simulink model "pure_linearization"  (R2023a)
settings: Solver=VariableStepAuto  StartTime=0.0  StopTime=5  RelTol=1e-3
settings Model: Creator=szymo  LastModifiedBy=szymo

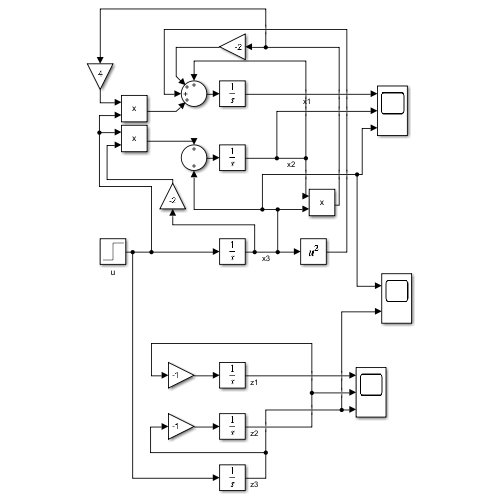
[thumbnail: Simulink's stored preview of the top-level diagram]
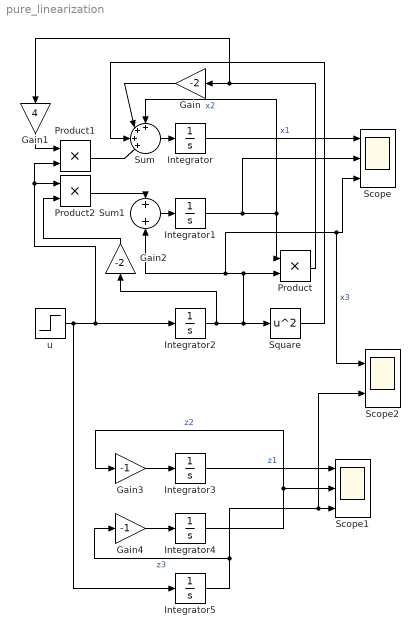
== system pure_linearization ==
  Gain : Gain  Gain=-2
  Gain1 : Gain  Gain=4
  Gain2 : Gain  Gain=-2
  Gain3 : Gain  Gain=-1
  Gain4 : Gain  Gain=-1
  Integrator{,1..5} (6 alike) : Integrator
  Product : Product
  Product1 : Product
  Product2 : Product
  Scope : Scope  NumInputPorts=3
  Scope1 : Scope  NumInputPorts=3
  Scope2 : Scope  NumInputPorts=2
  Square : Math  Operator=square
  Sum : Sum  Inputs=++++|
  Sum1 : Sum
  u : Step  Time=0  SampleTime=0
  wires:
  Sum/1 -> Integrator/1
  Integrator1/1 -> Scope/2, Product/1, Sum/1  "x2"
  Integrator/1 -> Scope/1  "x1"
  Integrator2/1 -> Gain2/1, Scope2/1, Scope/3, Sum1/2, Product/2, Square/1  "x3"
  Product/1 -> Gain1/1, Gain/1
  Gain/1 -> Sum/2
  Square/1 -> Sum/3
  Sum1/1 -> Integrator1/1
  u/1 -> Integrator5/1, Product2/1, Product1/2, Integrator2/1
  Product1/1 -> Sum/4
  Gain1/1 -> Product1/1
  Gain2/1 -> Product2/2
  Product2/1 -> Sum1/1
  Integrator3/1 -> Scope1/1  "z1"
  Integrator4/1 -> Scope1/2, Gain3/1  "z2"
  Integrator5/1 -> Scope2/2, Scope1/3, Gain4/1  "z3"
  Gain4/1 -> Integrator4/1
  Gain3/1 -> Integrator3/1
